simulink model "CRL_MCLV_V2_33EP256MC506_SlidingModeObserver_DualShunt_R2015a"  (R2015a)
settings: Solver=FixedStepDiscrete  StartTime=0.0  StopTime=10.0  FixedStep=.00005  RelTol=1e-3
PreLoadFcn:
  | UserParams;
values from neighbouring files (symbols this model uses):
  DELTA_STARTUP_RAMP = round( (MINSPEEDINRPM*POLEPAIRS*LOOPTIMEINSEC*LOOPTIMEINSEC*65536*65536/(60*OPENLOOPTIMEINSEC)) )    [UserParams.m]
  TS = LOOPTIMEINSEC    (= 5e-05)    [UserParams.m]
undefined symbols (not defined in the file or in its folder): A4, B15, B9, C5, C6, D8, F0, F1, Max, ms, P20, P41, P47, P53, P54, P96, P97, Pin, PWMmax, Resol, us
libraries: MCHP_Blockset x18, simulink x12
(part 2 of 2)

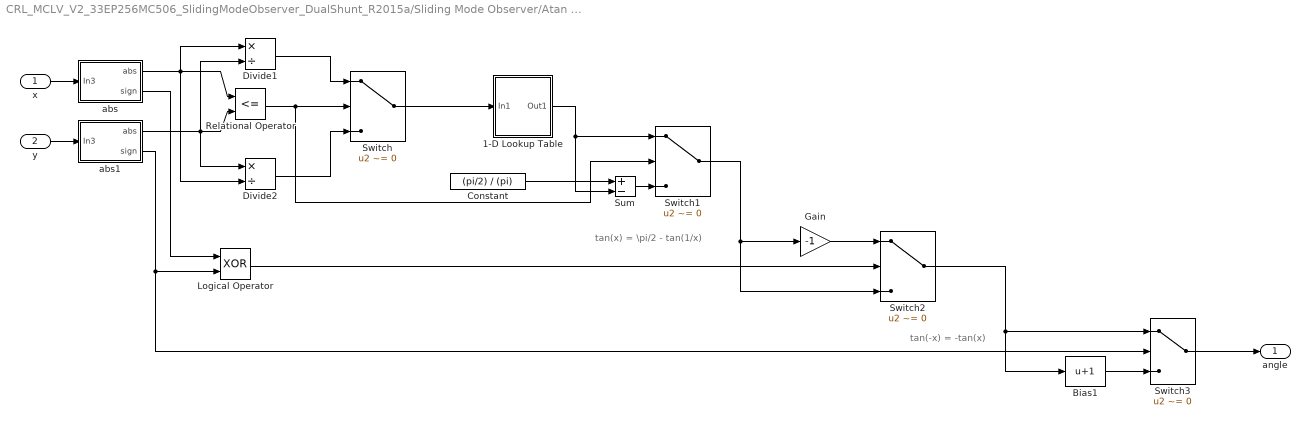
== system CRL_MCLV_V2_33EP256MC506_SlidingModeObserver_DualShunt_R2015a/Sliding Mode Observer/Atan x1 ==
  note: tan(x) = \pi/2 - tan(1/x)
  note: tan(-x) = -tan(x)
  x : Inport
  y : Inport  Port=2
  1-D Lookup Table : Subsystem  Description=Replaced Block  mask(Replaced Block){}
      mask help: This block has been replaced with an empty subsystem because it used functionality that is unavailable in Simulink R2015a.
      mask Display: fprintf('Replaced: %s\n','Lookup_n-D')
  Bias1 : Bias  Bias=1
  Constant : Constant  Value=(pi/2) / (pi)  OutDataTypeStr=Inherit: Inherit via back propagation
  Divide1 : Product  Inputs=*/  OutDataTypeStr=fixdt(0,16,15)
  Divide2 : Product  Inputs=*/  OutDataTypeStr=fixdt(0,16,15)
  Gain : Gain  Gain=-1  OutDataTypeStr=Inherit: Same as input
  Logical Operator : Logic  Operator=XOR  AllPortsSameDT=off  OutDataTypeStr=boolean
  Relational Operator : RelationalOperator  Operator=<=  OutDataTypeStr=boolean
  Sum : Sum  Inputs=+-
  Switch{,1..3} (4 alike) : Switch  Criteria=u2 ~= 0
  abs : Subsystem
  abs1 : Subsystem
  angle : Outport
  wires:
  Gain/1 -> Switch2/1
  Bias1/1 -> Switch3/3
  Switch3/1 -> angle/1
  Switch2/1 -> Switch3/1, Bias1/1
  Relational Operator/1 -> Switch/2, Switch1/2
  Divide2/1 -> Switch/3
  Divide1/1 -> Switch/1
  Switch/1 -> 1-D Lookup Table/1(In1)
  1-D Lookup Table/1(Out1) -> Switch1/1, Sum/2
  Constant/1 -> Sum/1
  Sum/1 -> Switch1/3
  abs/1(abs) -> Relational Operator/1, Divide1/1, Divide2/2
  x/1 -> abs/1(In3)
  abs1/1(abs) -> Relational Operator/2, Divide2/1, Divide1/2
  y/1 -> abs1/1(In3)
  abs/2(sign) -> Logical Operator/1
  abs1/2(sign) -> Logical Operator/2, Switch3/2
  Logical Operator/1 -> Switch2/2
  Switch1/1 -> Gain/1, Switch2/3

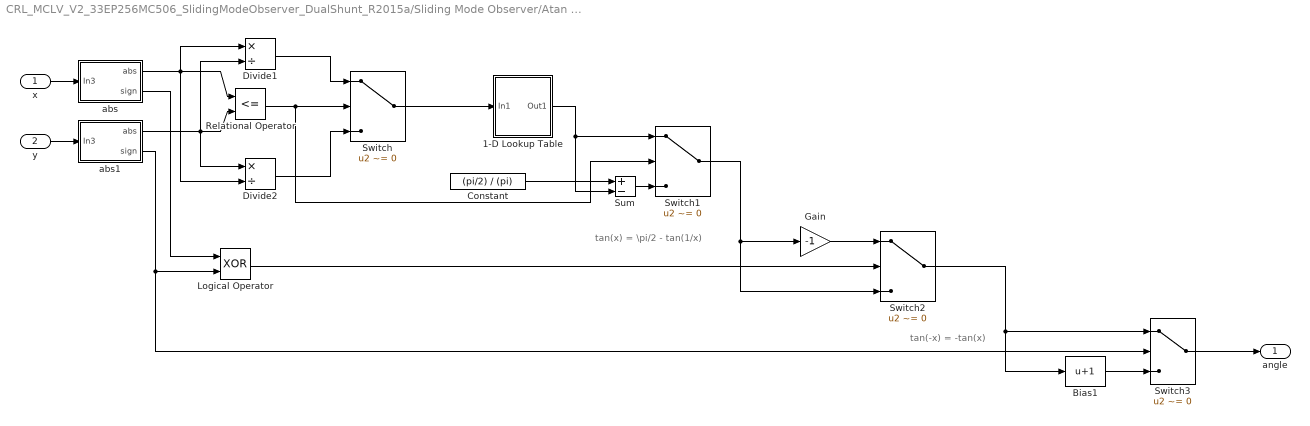
== system CRL_MCLV_V2_33EP256MC506_SlidingModeObserver_DualShunt_R2015a/Sliding Mode Observer/Atan x2 ==
  note: tan(-x) = -tan(x)
  note: tan(x) = \pi/2 - tan(1/x)
  x : Inport
  y : Inport  Port=2
  1-D Lookup Table : Subsystem  Description=Replaced Block  mask(Replaced Block){}
      mask help: This block has been replaced with an empty subsystem because it used functionality that is unavailable in Simulink R2015a.
      mask Display: fprintf('Replaced: %s\n','Lookup_n-D')
  Bias1 : Bias  Bias=1
  Constant : Constant  Value=(pi/2) / (pi)  OutDataTypeStr=Inherit: Inherit via back propagation
  Divide1 : Product  Inputs=*/  OutDataTypeStr=fixdt(0,16,15)
  Divide2 : Product  Inputs=*/  OutDataTypeStr=fixdt(0,16,15)
  Gain : Gain  Gain=-1  OutDataTypeStr=Inherit: Same as input
  Logical Operator : Logic  Operator=XOR  AllPortsSameDT=off  OutDataTypeStr=boolean
  Relational Operator : RelationalOperator  Operator=<=  OutDataTypeStr=boolean
  Sum : Sum  Inputs=+-
  Switch{,1..3} (4 alike) : Switch  Criteria=u2 ~= 0
  abs : Subsystem
  abs1 : Subsystem
  angle : Outport
  wires:
  Switch1/1 -> Switch2/3, Gain/1
  Logical Operator/1 -> Switch2/2
  abs1/2(sign) -> Switch3/2, Logical Operator/2
  abs/2(sign) -> Logical Operator/1
  y/1 -> abs1/1(In3)
  abs1/1(abs) -> Divide1/2, Divide2/1, Relational Operator/2
  x/1 -> abs/1(In3)
  abs/1(abs) -> Divide2/2, Divide1/1, Relational Operator/1
  Sum/1 -> Switch1/3
  Constant/1 -> Sum/1
  1-D Lookup Table/1(Out1) -> Sum/2, Switch1/1
  Switch/1 -> 1-D Lookup Table/1(In1)
  Divide1/1 -> Switch/1
  Divide2/1 -> Switch/3
  Relational Operator/1 -> Switch1/2, Switch/2
  Switch2/1 -> Bias1/1, Switch3/1
  Switch3/1 -> angle/1
  Bias1/1 -> Switch3/3
  Gain/1 -> Switch2/1

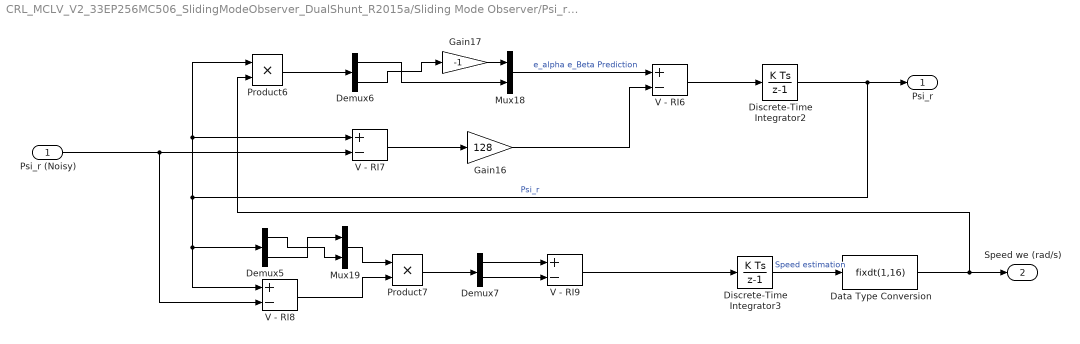
== system CRL_MCLV_V2_33EP256MC506_SlidingModeObserver_DualShunt_R2015a/Sliding Mode Observer/Psi_r Observer Speed Observer2 ==
  Psi_r (Noisy) : Inport
  Data Type Conversion : DataTypeConversion  OutMin=-5300 * 5 * (2*pi) / 60  OutMax=+5300 * 5 * (2*pi) / 60  OutDataTypeStr=fixdt(1,16)
  Demux5 : Demux  Outputs=2
  Demux6 : Demux  Outputs=2
  Demux7 : Demux  Outputs=2
  Discrete-Time Integrator2 : DiscreteIntegrator  gainval=1  SampleTime=-1  OutMin=-24  OutMax=24  OutDataTypeStr=fixdt(1,16)  UpperSaturationLimit=15  LowerSaturationLimit=-15
  Discrete-Time Integrator3 : DiscreteIntegrator  gainval=1000  SampleTime=-1  OutMin=-5300 * 5 * (2*pi) / 60  OutMax=5300 * 5 * (2*pi) / 60  OutDataTypeStr=fixdt(1,32)  RndMeth=Simplest  StateIdentifier=Speed
  Gain16 : Gain  Gain=128  OutMin=[-24*2*128]  OutMax=[24*2*128]  OutDataTypeStr=fixdt(1,16)
  Gain17 : Gain  Gain=-1  OutDataTypeStr=Inherit: Same as input
  Mux18 : Mux  Inputs=2
  Mux19 : Mux  Inputs=2
  Product6 : Product  OutDataTypeStr=fixdt(1,32,12)  SaturateOnIntegerOverflow=on  RndMeth=Zero
  Product7 : Product  OutMin=[-24*24]  OutMax=24*24  OutDataTypeStr=fixdt(1,16)  RndMeth=Simplest  SaturateOnIntegerOverflow=on
  V - RI6 : Sum  Inputs=+-  OutDataTypeStr=Inherit: Same as accumulator
  V - RI7 : Sum  Inputs=+-  OutMin=[-24*2]  OutMax=[24*2]  OutDataTypeStr=fixdt(1,16)
  V - RI8 : Sum  Inputs=+-  OutDataTypeStr=Inherit: Same as accumulator  RndMeth=Simplest  SaturateOnIntegerOverflow=on
  V - RI9 : Sum  Inputs=+-  OutMin=[-24*24*2]  OutMax=[-24*24*2]  OutDataTypeStr=fixdt(1,16)  RndMeth=Simplest  SaturateOnIntegerOverflow=on  InputSameDT=on
  Psi_r : Outport
  Speed we (rad/s) : Outport  Port=2
  wires:
  Gain16/1 -> V - RI6/2
  Discrete-Time Integrator2/1 -> Demux5/1, V - RI8/1, V - RI7/1, Product6/1, Psi_r/1  "Psi_r"
  Demux5/1 -> Mux19/2
  Demux6/2 -> Gain17/1
  Data Type Conversion/1 -> Speed we (rad/s)/1, Product6/2
  Psi_r (Noisy)/1 -> V - RI7/2, V - RI8/2
  Demux6/1 -> Mux18/2
  Discrete-Time Integrator3/1 -> Data Type Conversion/1  "Speed estimation"
  Gain17/1 -> Mux18/1
  Product6/1 -> Demux6/1
  Demux7/2 -> V - RI9/2
  Demux7/1 -> V - RI9/1
  Product7/1 -> Demux7/1
  V - RI8/1 -> Product7/2
  Mux19/1 -> Product7/1
  Demux5/2 -> Mux19/1
  Mux18/1 -> V - RI6/1  "e_alpha e_Beta Prediction"
  V - RI7/1 -> Gain16/1
  V - RI6/1 -> Discrete-Time Integrator2/1
  V - RI9/1 -> Discrete-Time Integrator3/1

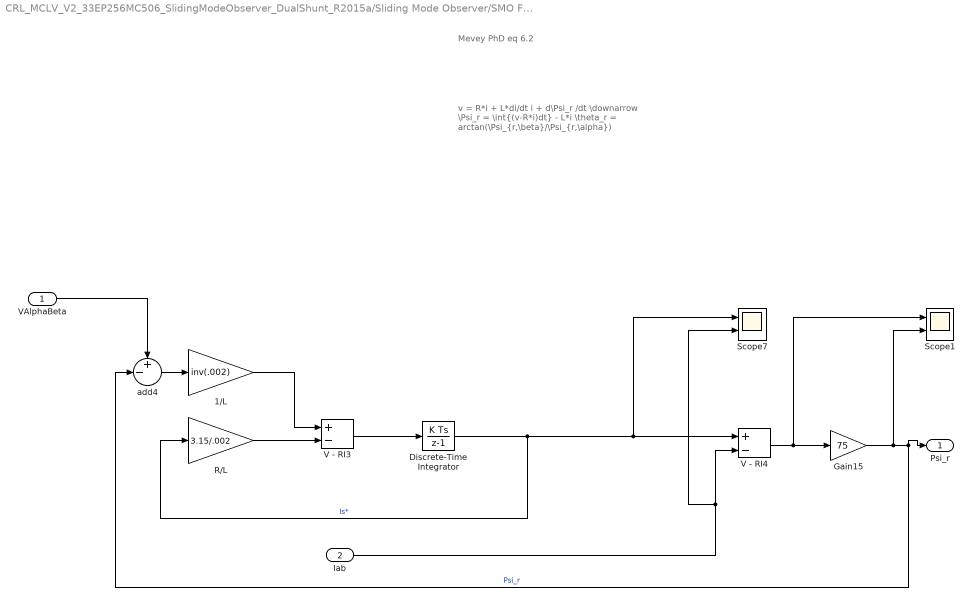
== system CRL_MCLV_V2_33EP256MC506_SlidingModeObserver_DualShunt_R2015a/Sliding Mode Observer/SMO FxPt ==
  note: Mevey PhD eq 6.2
  note: v = R*i + L*di/dt i + d\Psi_r /dt
      | \downarrow
      | \Psi_r = \int{(v-R*i)dt} - L*i
      | \theta_r = arctan(\Psi_{r,\beta}/\Psi_{r,\alpha})
  VAlphaBeta : Inport
  Iab : Inport  Port=2
  1/L : Gain  Gain=inv(.002)  OutMin=[-24] * inv(.002) *2  OutMax=[24] * inv(.002) *2  OutDataTypeStr=fixdt(1,16)
  Discrete-Time Integrator : DiscreteIntegrator  SampleTime=-1  OutMin=[-4.4]  OutMax=[4.4]  OutDataTypeStr=fixdt(1,16)
  Gain15 : Gain  Gain=75  OutMin=[-24]  OutMax=[24]  OutDataTypeStr=fixdt(1,16)  SaturateOnIntegerOverflow=on
  R/L : Gain  Gain=3.15/.002  OutMin=[-4.4] * 3.15/.002  OutMax=[4.4] * 3.15/.002  OutDataTypeStr=fixdt(1,16)
  Scope1 : Scope  NumInputPorts=2
      settings: YMin=-39.99988~-5  YMax=39.9989~5
  Scope7 : Scope  NumInputPorts=2
      settings: TimeRange=5  YMin=-3.23778~-5  YMax=3.35877~5  SaveName=ScopeData6
  V - RI3 : Sum  Inputs=+-  OutDataTypeStr=Inherit: Same as accumulator
  V - RI4 : Sum  Inputs=+-  OutDataTypeStr=Inherit: Same as accumulator
  add4 : Sum  Inputs=+-|  OutDataTypeStr=Inherit: Same as accumulator  SaturateOnIntegerOverflow=on
  Psi_r : Outport
  wires:
  1/L/1 -> V - RI3/1
  R/L/1 -> V - RI3/2
  add4/1 -> 1/L/1
  VAlphaBeta/1 -> add4/1
  V - RI3/1 -> Discrete-Time Integrator/1
  Discrete-Time Integrator/1 -> V - RI4/1, Scope7/1, R/L/1  "Is*"
  V - RI4/1 -> Scope1/1, Gain15/1
  Iab/1 -> V - RI4/2, Scope7/2
  Gain15/1 -> Scope1/2, add4/2, Psi_r/1  "Psi_r"

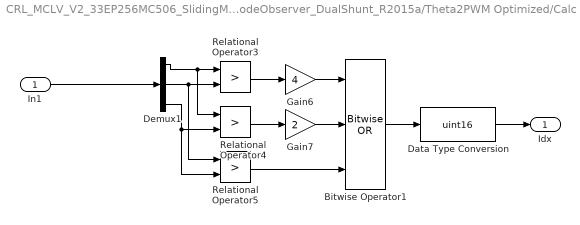
== system CRL_MCLV_V2_33EP256MC506_SlidingModeObserver_DualShunt_R2015a/Theta2PWM Optimized/Calc Index ==
  In1 : Inport
  Bitwise Operator1 : simulink/Logic and Bit Operations/Bitwise Operator  logicop=OR  UseBitMask=off  NumInputPorts=3  BitMask=bin2dec('11011001')  BitMaskRealWorld=Stored Integer
  Data Type Conversion : DataTypeConversion  OutDataTypeStr=uint16  ConvertRealWorld=Stored Integer (SI)
  Demux1 : Demux  Outputs=3
  Gain6 : Gain  Gain=4  OutDataTypeStr=Inherit: Same as input
  Gain7 : Gain  Gain=2  OutDataTypeStr=Inherit: Same as input
  Relational Operator3 : RelationalOperator  Operator=>  OutDataTypeStr=fixdt(1,16)
  Relational Operator4 : RelationalOperator  Operator=>  OutDataTypeStr=fixdt(1,16)
  Relational Operator5 : RelationalOperator  Operator=>  OutDataTypeStr=fixdt(1,16)
  Idx : Outport
  wires:
  Gain7/1 -> Bitwise Operator1/2
  Gain6/1 -> Bitwise Operator1/1
  Relational Operator5/1 -> Bitwise Operator1/3
  Relational Operator3/1 -> Gain6/1
  Demux1/2 -> Relational Operator5/1, Relational Operator3/2
  Demux1/3 -> Relational Operator5/2, Relational Operator4/2
  Relational Operator4/1 -> Gain7/1
  Demux1/1 -> Relational Operator4/1, Relational Operator3/1
  Bitwise Operator1/1 -> Data Type Conversion/1
  In1/1 -> Demux1/1
  Data Type Conversion/1 -> Idx/1

== system CRL_MCLV_V2_33EP256MC506_SlidingModeObserver_DualShunt_R2015a/Theta2PWM Optimized/Maximum Duty-Cycle ==
  In1 : Inport
  Constant1 : Constant  Value=PWMmax  OutDataTypeStr=uint16
  MinMax1 : MinMax  Function=max  OutDataTypeStr=int16  InputSameDT=on
  Sum1 : Sum  Inputs=+-  AccumDataTypeStr=uint16  OutDataTypeStr=Inherit: Same as accumulator  RndMeth=Simplest
  Sum2 : Sum  Inputs=|++  AccumDataTypeStr=uint16  OutDataTypeStr=Inherit: Same as accumulator  RndMeth=Simplest
  Out1 : Outport
  wires:
  Sum1/1 -> Sum2/2
  Sum2/1 -> Out1/1
  In1/1 -> MinMax1/1, Sum2/1
  MinMax1/1 -> Sum1/2
  Constant1/1 -> Sum1/1

== system CRL_MCLV_V2_33EP256MC506_SlidingModeObserver_DualShunt_R2015a/Theta2PWM Optimized/Minimum Duty-Cycle ==
  In1 : Inport
  Bias : Bias  Bias=-round( (2e-6/5e-5) *PWMmax )
  MinMax1 : MinMax  OutDataTypeStr=int16  InputSameDT=on
  Sum2 : Sum  Inputs=|+-  AccumDataTypeStr=uint16  OutDataTypeStr=Inherit: Same as accumulator  RndMeth=Simplest
  Out1 : Outport
  wires:
  Bias/1 -> Sum2/2
  MinMax1/1 -> Bias/1
  Sum2/1 -> Out1/1
  In1/1 -> Sum2/1, MinMax1/1

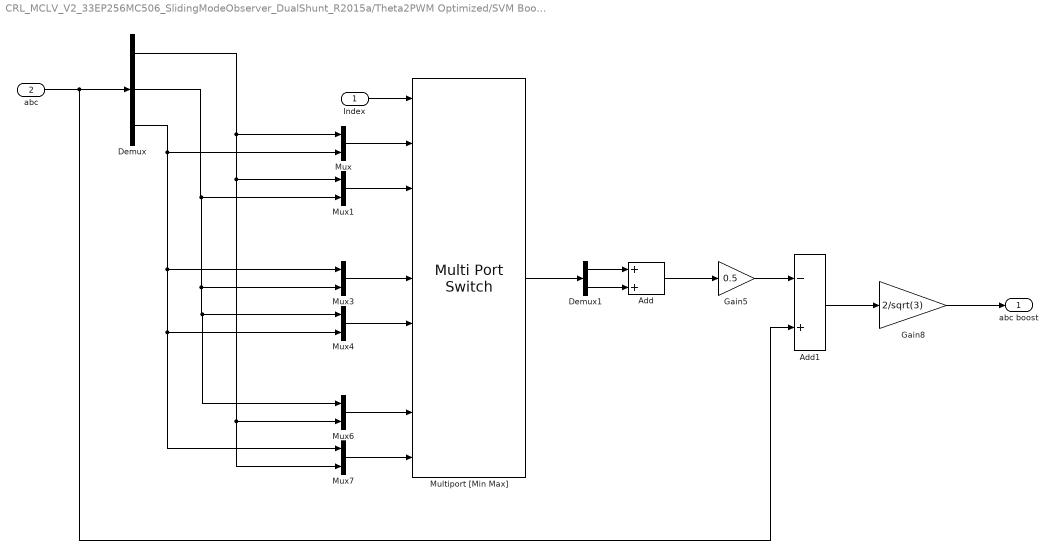
== system CRL_MCLV_V2_33EP256MC506_SlidingModeObserver_DualShunt_R2015a/Theta2PWM Optimized/SVM Boost ==
  Index : Inport
  abc : Inport  Port=2
  Add : Sum  OutDataTypeStr=Inherit: Same as accumulator  RndMeth=Simplest
  Add1 : Sum  Inputs=-+  OutDataTypeStr=Inherit: Same as accumulator  RndMeth=Simplest
  Demux : Demux  Outputs=3
  Demux1 : Demux  Outputs=2
  Gain5 : Gain  Gain=0.5  RndMeth=Simplest  OutDataTypeStr=Inherit: Same as input
  Gain8 : Gain  Gain=2/sqrt(3)  RndMeth=Simplest  OutDataTypeStr=Inherit: Same as input
  Multiport [Min Max] : MultiPortSwitch  DataPortOrder=Zero-based contiguous  Inputs=8  DiagnosticForDefault=None
  Mux{,1,3..4,6..7} (6 alike) : Mux  Inputs=2
  abc boost : Outport
  wires:
  Demux1/2 -> Add/2
  Demux1/1 -> Add/1
  Multiport [Min Max]/1 -> Demux1/1
  Demux/2 -> Mux1/2, Mux3/2, Mux4/1, Mux6/1
  Demux/3 -> Mux7/1, Mux4/2, Mux3/1, Mux/2
  Demux/1 -> Mux/1, Mux1/1, Mux6/2, Mux7/2
  Mux7/1 -> Multiport [Min Max]/9
  Mux6/1 -> Multiport [Min Max]/8
  Mux4/1 -> Multiport [Min Max]/6
  Mux3/1 -> Multiport [Min Max]/5
  Mux1/1 -> Multiport [Min Max]/3
  Mux/1 -> Multiport [Min Max]/2
  Index/1 -> Multiport [Min Max]/1
  Gain8/1 -> abc boost/1
  abc/1 -> Demux/1, Add1/2
  Add1/1 -> Gain8/1
  Gain5/1 -> Add1/1
  Add/1 -> Gain5/1

== system CRL_MCLV_V2_33EP256MC506_SlidingModeObserver_DualShunt_R2015a/Theta2PWM Optimized/Sine Simpler ==
  note: Gain is about 2us (70 MIPS)
  Theta : Inport
  Bias1 : Bias  Bias=0.25
  Look-Up Table (sin) : Subsystem  Description=Replaced Block  mask(Replaced Block){}
      mask help: This block has been replaced with an empty subsystem because it used functionality that is unavailable in Simulink R2015a.
      mask Display: fprintf('Replaced: %s\n','Lookup_n-D')
  Look-Up Table (sin)1 : Subsystem  Description=Replaced Block  mask(Replaced Block){}
      mask help: This block has been replaced with an empty subsystem because it used functionality that is unavailable in Simulink R2015a.
      mask Display: fprintf('Replaced: %s\n','Lookup_n-D')
  Sine1 : simulink/Lookup Tables/Sine  Formula=sin(2*pi*u) and cos(2*pi*u)  NumDataPoints=(2^5)+1  OutputWordLength=16  InternalRulePriority=Speed
  cos(2*pi*u) : Outport
  sin(2*pi*u) : Outport  Port=2
  wires:
  Bias1/1 -> Look-Up Table (sin)1/1(In1)
  Theta/1 -> Bias1/1, Look-Up Table (sin)/1(In1), Sine1/1
  Look-Up Table (sin)/1(Out1) -> sin(2*pi*u)/1
  Look-Up Table (sin)1/1(Out1) -> cos(2*pi*u)/1

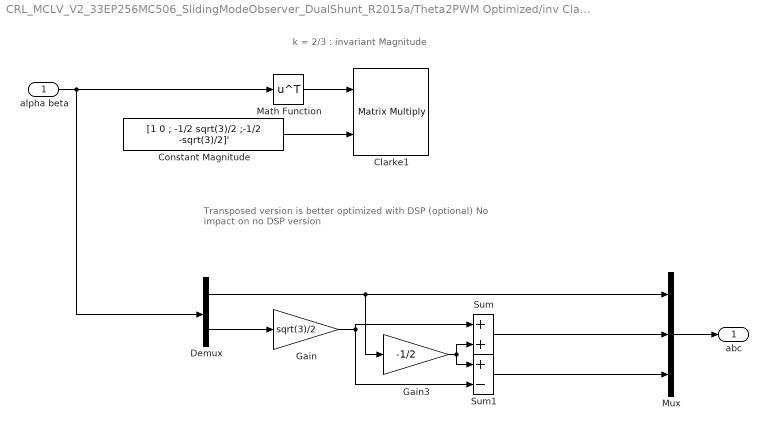
== system CRL_MCLV_V2_33EP256MC506_SlidingModeObserver_DualShunt_R2015a/Theta2PWM Optimized/inv Clark ==
  note: k = 2/3 : invariant Magnitude
  note: Transposed version is better optimized with DSP (optional)
      | No impact on no DSP version
  alpha beta : Inport
  Clarke1 : Product  Multiplication=Matrix(*)  RndMeth=Convergent  OutDataTypeStr=Inherit: Same as first input
  Constant Magnitude : Constant  Value=[1 0 ; -1/2 sqrt(3)/2 ;-1/2 -sqrt(3)/2]'  OutDataTypeStr=Inherit: Inherit via back propagation  SampleTime=-1
  Demux : Demux  Outputs=2
  Gain : Gain  Gain=sqrt(3)/2  OutDataTypeStr=Inherit: Same as input
  Gain3 : Gain  Gain=-1/2  RndMeth=Simplest  OutDataTypeStr=Inherit: Same as input
  Math Function : Math  Operator=transpose  SaturateOnIntegerOverflow=on
  Mux : Mux  Inputs=3
  Sum : Sum  RndMeth=Simplest  OutDataTypeStr=Inherit: Same as first input
  Sum1 : Sum  Inputs=+-  RndMeth=Simplest  OutDataTypeStr=Inherit: Same as first input
  abc : Outport
  wires:
  Gain3/1 -> Sum/2, Sum1/1
  Sum1/1 -> Mux/3
  Sum/1 -> Mux/2
  Gain/1 -> Sum1/2, Sum/1
  Demux/2 -> Gain/1
  Demux/1 -> Mux/1, Gain3/1
  Math Function/1 -> Clarke1/1
  alpha beta/1 -> Math Function/1, Demux/1
  Constant Magnitude/1 -> Clarke1/2
  Mux/1 -> abc/1

== system CRL_MCLV_V2_33EP256MC506_SlidingModeObserver_DualShunt_R2015a/DUAL SHUNT Center Aligned/MOTOR - Board Sensor/encoder scaled ==
  Rst : Inport
  Direct Lookup Table (n-D) : LookupNDDirect  NumberOfTableDimensions=1  Table=[0:199]*inv(200)  TableDataTypeStr=fixdt(0,16,16)
      settings: LockScale=on
  Q0.4 : DataTypeConversion
  QEI : MCHP_Blockset/QEI/QEI  QEI_REF=1  QEI_MODE=Quadrature Encoder  QEI_x2mode=off  QEI_PulseCountDir=Down  PIN_QEA=Dynamic Options  PIN_QEA_TXT=C6 / P54 / Pin[50]  PIN_QEB=Dynamic Options  PIN_QEB_TXT=F0 / P96 / Pin[58]  SWPAB=on  QEAPOL=off  QEBPOL=off  SampleTime=-1  INDXxCNT_Output=is not an output  POSxCNT_Output=is a 16 bits unsigned block output  RESET_Input=on  PIMOD_mode=position is cyclique between user defined boundaries  PIMOD_modeB=Never reset position  PIMOD_reset=on next INDEX event  PIN_INDEX=Dynamic Options  PIN_INDEX_TXT=B15 / P47 / Pin[3]  IMV=QEA = 1 and QEB = 0  IMV_x2=QEA = 1  PIN_HOME=Dynamic Options  PIN_HOME_TXT=B9 / P41 / Pin[49]  QEIxLEC_GEC=[0 199]  QEIxIC=0  PCIIRQ=off  IDXPOL=off  HOMPOL=on  VELxCNT_Output=is not an output  INTxHLD_Output=is not an output  MaxPeriod=0.1  FILTREN=on  QFDIV_popup=Dynamic Options  QFDIV_popup_TXT=364.58 kHz  FILTER_CutOffFreq=100e3  PIN_CCMP=Dynamic Options  PIN_CCMP_TXT=A4 / P20 / Pin[33]  MCHP_PORT={QEI1 A}{QEA1}5:0:P54;{QEI1 B}{QEB1}5:0:P96;  MCHP_MASTERLINK=CRL_MCLV_V2_33EP256MC506_SlidingModeObserver_DualShunt_R2015a/Microchip Master  QEI_IntPri=5
  Rate Transition4 : RateTransition  X0=1
  theta_enc_fract : Outport
  wires:
  Rate Transition4/1 -> QEI/1
  Q0.4/1 -> Rate Transition4/1
  Rst/1 -> Q0.4/1
  Direct Lookup Table (n-D)/1 -> theta_enc_fract/1
  QEI/1 -> Direct Lookup Table (n-D)/1

== system CRL_MCLV_V2_33EP256MC506_SlidingModeObserver_DualShunt_R2015a/Sliding Mode Observer/Atan x1/1-D Lookup Table ==
  In1 : Inport
  Ground1 : Ground
  Terminator1 : Terminator
  Out1 : Outport
  wires:
  Ground1/1 -> Out1/1
  In1/1 -> Terminator1/1

== system CRL_MCLV_V2_33EP256MC506_SlidingModeObserver_DualShunt_R2015a/Sliding Mode Observer/Atan x1/abs ==
  In3 : Inport
  Compare To Zero : simulink/Logic and Bit Operations/Compare To Zero  relop=>=  OutDataTypeStr=boolean
  Gain : Gain  Gain=-1  OutDataTypeStr=Inherit: Same as input
  Switch2 : Switch  Criteria=u2 ~= 0
  abs : Outport
  sign : Outport  Port=2
  wires:
  Compare To Zero/1 -> Switch2/2, sign/1
  In3/1 -> Compare To Zero/1, Switch2/1, Gain/1
  Gain/1 -> Switch2/3
  Switch2/1 -> abs/1

== system CRL_MCLV_V2_33EP256MC506_SlidingModeObserver_DualShunt_R2015a/Sliding Mode Observer/Atan x1/abs1 ==
  In3 : Inport
  Compare To Zero : simulink/Logic and Bit Operations/Compare To Zero  relop=>=  OutDataTypeStr=boolean
  Gain : Gain  Gain=-1  OutDataTypeStr=Inherit: Same as input
  Switch2 : Switch  Criteria=u2 ~= 0
  abs : Outport
  sign : Outport  Port=2
  wires:
  Switch2/1 -> abs/1
  Gain/1 -> Switch2/3
  In3/1 -> Gain/1, Switch2/1, Compare To Zero/1
  Compare To Zero/1 -> sign/1, Switch2/2

== system CRL_MCLV_V2_33EP256MC506_SlidingModeObserver_DualShunt_R2015a/Sliding Mode Observer/Atan x2/1-D Lookup Table ==
  In1 : Inport
  Ground1 : Ground
  Terminator1 : Terminator
  Out1 : Outport
  wires:
  Ground1/1 -> Out1/1
  In1/1 -> Terminator1/1

== system CRL_MCLV_V2_33EP256MC506_SlidingModeObserver_DualShunt_R2015a/Sliding Mode Observer/Atan x2/abs ==
  In3 : Inport
  Compare To Zero : simulink/Logic and Bit Operations/Compare To Zero  relop=>=  OutDataTypeStr=boolean
  Gain : Gain  Gain=-1  OutDataTypeStr=Inherit: Same as input
  Switch2 : Switch  Criteria=u2 ~= 0
  abs : Outport
  sign : Outport  Port=2
  wires:
  Switch2/1 -> abs/1
  Gain/1 -> Switch2/3
  In3/1 -> Gain/1, Switch2/1, Compare To Zero/1
  Compare To Zero/1 -> sign/1, Switch2/2

== system CRL_MCLV_V2_33EP256MC506_SlidingModeObserver_DualShunt_R2015a/Sliding Mode Observer/Atan x2/abs1 ==
  In3 : Inport
  Compare To Zero : simulink/Logic and Bit Operations/Compare To Zero  relop=>=  OutDataTypeStr=boolean
  Gain : Gain  Gain=-1  OutDataTypeStr=Inherit: Same as input
  Switch2 : Switch  Criteria=u2 ~= 0
  abs : Outport
  sign : Outport  Port=2
  wires:
  Compare To Zero/1 -> Switch2/2, sign/1
  In3/1 -> Compare To Zero/1, Switch2/1, Gain/1
  Gain/1 -> Switch2/3
  Switch2/1 -> abs/1

== system CRL_MCLV_V2_33EP256MC506_SlidingModeObserver_DualShunt_R2015a/Theta2PWM Optimized/Sine Simpler/Look-Up Table (sin) ==
  In1 : Inport
  Ground1 : Ground
  Terminator1 : Terminator
  Out1 : Outport
  wires:
  Ground1/1 -> Out1/1
  In1/1 -> Terminator1/1

== system CRL_MCLV_V2_33EP256MC506_SlidingModeObserver_DualShunt_R2015a/Theta2PWM Optimized/Sine Simpler/Look-Up Table (sin)1 ==
  In1 : Inport
  Ground1 : Ground
  Terminator1 : Terminator
  Out1 : Outport
  wires:
  Ground1/1 -> Out1/1
  In1/1 -> Terminator1/1
